simulink model "SystemSISOC"  (Simulink 10.0)
settings: Solver=ode45  StartTime=0.0  StopTime=tend  MaxStep=0.01  RelTol=1e-3  EnableMultiTasking=on
InitFcn:
  | global p p1 P P1;
values from neighbouring files (symbols this model uses):
  p1 = p    [Blok_identyfikacji_zad_3.m]    (also in Zad_1_1.m = p_; Zad_1_1_8_kolorowe.m = p_; Zad_3_1.m)
  sigma2e = 0.1    [Zad_3_1.m]
  Tf = 8*Tp    (= 0.4)    [Zad_3_1.m]
  Tp = 0.1    [ZADANIE_1_2.m]    (also in ZADANIE_2_1.m; Zad_1_1.m; Zad_1_1_8_kolorowe.m; Zad_2_1_zapominanie.m)
libraries: simulink x1
settings Model: Creator=mgmil  LastModifiedBy=mgmil
settings DataIOCC: LimitDataPoints=on  SignalLoggingSaveFormat=ModelDataLogs
settings OptimizationCC: InitFltsAndDblsToZero=on
settings DebuggingCC: SaveWithParameterizedLinksMsg=none  SignalResolutionControl=TryResolveAllWithWarning  SolverPrmCheckMsg=warning  MultiTaskDSMMsg=warning  MultiTaskCondExecSysMsg=none  FcnCallInpInsideContextMsg=warning
settings SFSimCC: SimUseLocalCustomCode=on  CustomCodeUndefinedFunction=FilterOut
settings RTWCC: RTWUseLocalCustomCode=on
settings GRTTargetCC: TargetFcnLib=ansi_tfl_tmw.mat

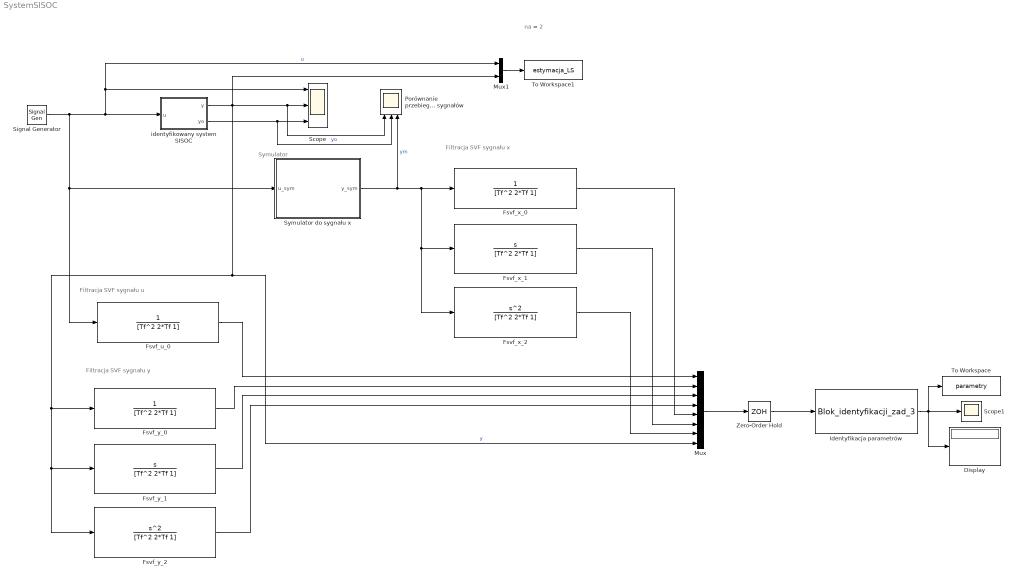
== system SystemSISOC ==
  note: Symulator
  note: Filtracja SVF sygnału y
  note: Filtracja SVF sygnału u
  note: na = 2
  note: Filtracja SVF sygnału x
  Display : Display
  Fsvf_u_0 : TransferFcn  Numerator=1  Denominator=[Tf^2 2*Tf 1]
  Fsvf_x_0 : TransferFcn  Numerator=1  Denominator=[Tf^2 2*Tf 1]
  Fsvf_x_1 : TransferFcn  Numerator=[1 0]  Denominator=[Tf^2 2*Tf 1]
  Fsvf_x_2 : TransferFcn  Numerator=[1 0 0]  Denominator=[Tf^2 2*Tf 1]
  Fsvf_y_0 : TransferFcn  Numerator=1  Denominator=[Tf^2 2*Tf 1]
  Fsvf_y_1 : TransferFcn  Numerator=[1 0]  Denominator=[Tf^2 2*Tf 1]
  Fsvf_y_2 : TransferFcn  Numerator=[1 0 0]  Denominator=[Tf^2 2*Tf 1]
  Identyfikacja parametrów : MATLABFcn  MATLABFcn=Blok_identyfikacji_zad_3
  Mux : Mux  Inputs=8
  Mux1 : Mux  Inputs=2
  Porównanie przebiegów sygnałów : Scope  NumInputPorts=3
  Scope : Scope  NumInputPorts=3
  Scope1 : Scope
  Signal Generator : SignalGenerator  WaveForm=square  Frequency=0.04
  Symulator do sygnału x : Subsystem
  To Workspace : ToWorkspace  VariableName=parametry  SampleTime=-1
  To Workspace1 : ToWorkspace  VariableName=estymacja_LS  SampleTime=-1
  Zero-Order Hold : ZeroOrderHold  SampleTime=Tp
  identyfikowany system SISOC : Subsystem
  wires:
  Signal Generator/1 -> Scope/1, Mux1/1, identyfikowany system SISOC/1(u), Symulator do sygnału x/1("u_sym "), Fsvf_u_0/1  "u"
  identyfikowany system SISOC/1(y) -> Mux/8, Fsvf_y_0/1, Fsvf_y_1/1, Fsvf_y_2/1, Mux1/2, Scope/2, Porównanie przebiegów sygnałów/1  "y"
  identyfikowany system SISOC/2(yo) -> Porównanie przebiegów sygnałów/2, Scope/3  "yo"
  Symulator do sygnału x/1(y_sym) -> Fsvf_x_2/1, Fsvf_x_1/1, Fsvf_x_0/1, Porównanie przebiegów sygnałów/3  "ym"
  Fsvf_u_0/1 -> Mux/1
  Fsvf_y_0/1 -> Mux/2
  Fsvf_y_1/1 -> Mux/3
  Fsvf_y_2/1 -> Mux/4
  Fsvf_x_0/1 -> Mux/5
  Fsvf_x_1/1 -> Mux/6
  Fsvf_x_2/1 -> Mux/7
  Identyfikacja parametrów/1 -> Display/1, To Workspace/1, Scope1/1
  Mux1/1 -> To Workspace1/1
  Zero-Order Hold/1 -> Identyfikacja parametrów/1
  Mux/1 -> Zero-Order Hold/1

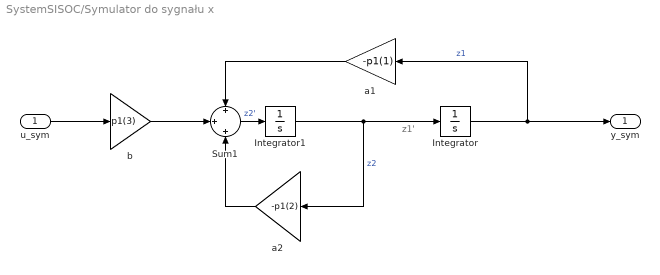
== system SystemSISOC/Symulator do sygnału x ==
  note: z1'
  "u_sym " : Inport
  Integrator : Integrator
  Integrator1 : Integrator
  Sum1 : Sum  Inputs=+|+|+
  a1 : Gain  Gain=-p1(1)
  a2 : Gain  Gain=-p1(2)
  b : Gain  Gain=p1(3)
  y_sym : Outport
  wires:
  Integrator/1 -> a1/1, y_sym/1  "z1"
  "u_sym "/1 -> b/1
  Sum1/1 -> Integrator1/1  "z2'"
  Integrator1/1 -> Integrator/1, a2/1  "z2"
  a2/1 -> Sum1/3
  a1/1 -> Sum1/1
  b/1 -> Sum1/2

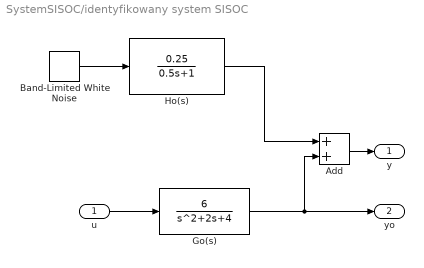
== system SystemSISOC/identyfikowany system SISOC ==
  u : Inport
  Add : Sum
  Band-Limited White Noise : simulink/Sources/Band-Limited White Noise  Cov=[sigma2e]  Ts=Tp*0.1  seed=[2941]
  Go(s) : TransferFcn  Numerator=[6]  Denominator=[1 2 4]
  Ho(s) : TransferFcn  Numerator=[0.25]  Denominator=[0.5 1]
  y : Outport
  yo : Outport  Port=2
  wires:
  Band-Limited White Noise/1 -> Ho(s)/1
  Ho(s)/1 -> Add/1
  Go(s)/1 -> Add/2, yo/1
  Add/1 -> y/1
  u/1 -> Go(s)/1
